simulink library "tire"  (R2020b)
settings: Solver=VariableStepAuto  StartTime=0.0  StopTime=10.0  RelTol=1e-3
undefined symbols (not defined in the file or in its folder): MF_coeff, tire_data
libraries: RF_transformations x6, Resettable_Unit_Delay x4, $bdroot x4, Resettable_Derivative x2, simulink x1, Resettable_Integrator x1
(part 2 of 2)

== matlab function tire/My_Tire_programmable/Gyroscopic couple ==
  data: Omega input; Mz_gyr output; Re input; Fz input; dvdt input; tire_data parameter; USE_MODE parameter
function Mz_gyr = fcn(Omega, Re, Fz, dvdt, tire_data, USE_MODE)

% Mz due to the gyroscopic effect of the yre belt deflections (7.2.5 Book)

parsed_um = dec2base(abs(USE_MODE),10) - '0';
parsed_um = [zeros(1,2-length(parsed_um)),parsed_um];
USE_MODE_1    = parsed_um(2);          % type of calculation

if USE_MODE_1 == 2 || USE_MODE_1 == 3 || USE_MODE_1 == 4 || USE_MODE_1 == 5  
    c_gyr = 0.5; % for a radial ply steel-belted car tire,
    m_t = tire_data.BELT_MASS;
    Fz_0 = tire_data.FNOMIN;
    
    Mz_gyr = c_gyr * m_t * Re * Omega * dvdt * Fz/Fz_0 ;
else
    Mz_gyr = 0;
end

== matlab function tire/My_Tire/Fz ==
  data: rho input; rho_dot input; F_x input; F_y input; omega input; gamma input; p_i input; Fz output; tire_data parameter; USE_MODE parameter; Fz_flag parameter
function Fz = fcn(rho,rho_dot,F_x,F_y,omega,gamma,p_i,tire_data, USE_MODE, Fz_flag)

% !! rho take the value of external Fz in case of Fz_flag ~= 0

if Fz_flag == 0
    % initialize tire class !!! TEMPORARY WORKAROUND !!!
    if tire_data.FITTYP == 62
        TIRE = pacejka_model_62_class(tire_data, USE_MODE);
        Fz = TIRE.compute_F_z(rho, rho_dot, omega, gamma, p_i, F_x, F_y);
    elseif tire_data.FITTYP == 52
        TIRE = pacejka_model_52_class(tire_data, USE_MODE);
        Fz = TIRE.compute_F_z(rho, rho_dot, omega, gamma, p_i, F_x, F_y);
    else
        Fz = NaN;
    end
    
else
    Fz = rho; % Fz passtrough
end
end

== matlab function tire/My_Tire_programmable/MATLAB Function ==
  data: phi_t input; sigma_k output; F_z input; tire_p input; sigma_a output; tire_data parameter; USE_MODE parameter; sigma_p output
function [sigma_k, sigma_a, sigma_p] = calcRelax(phi_t, F_z, tire_p, tire_data, USE_MODE)

% initialize tire class !!! TEMPORARY WORKAROUND !!! 
if tire_data.FITTYP == 62
    TIRE = pacejka_model_62_class(tire_data, USE_MODE);
    [sigma_k, sigma_a, sigma_p] = TIRE.compute_relax( phi_t, F_z, tire_p);
elseif tire_data.FITTYP == 52
    TIRE = pacejka_model_52_class(tire_data, USE_MODE);
    [sigma_k, sigma_a, sigma_p] = TIRE.compute_relax( phi_t, F_z, tire_p);
else
    sigma_k = NaN;
    sigma_a = NaN;
    sigma_p = NaN;
end
